simulink model "TailSitter_waypoints_continuous"  (R2018b)
settings: Solver=VariableStepAuto  StartTime=0.0  StopTime=400  RelTol=1e-3
values from neighbouring files (symbols this model uses):
  p =     [ds.mat]    (also in vxs.mat)
undefined symbols (not defined in the file or in its folder): quatnormalize
libraries: aerolibutil x18, simulink x6, sharedutil x3, vrlib x2, simulink_extras x2, sharedtransform x1
(part 1 of 4)
settings Model: Creator=Robert  LastModifiedBy=Robert

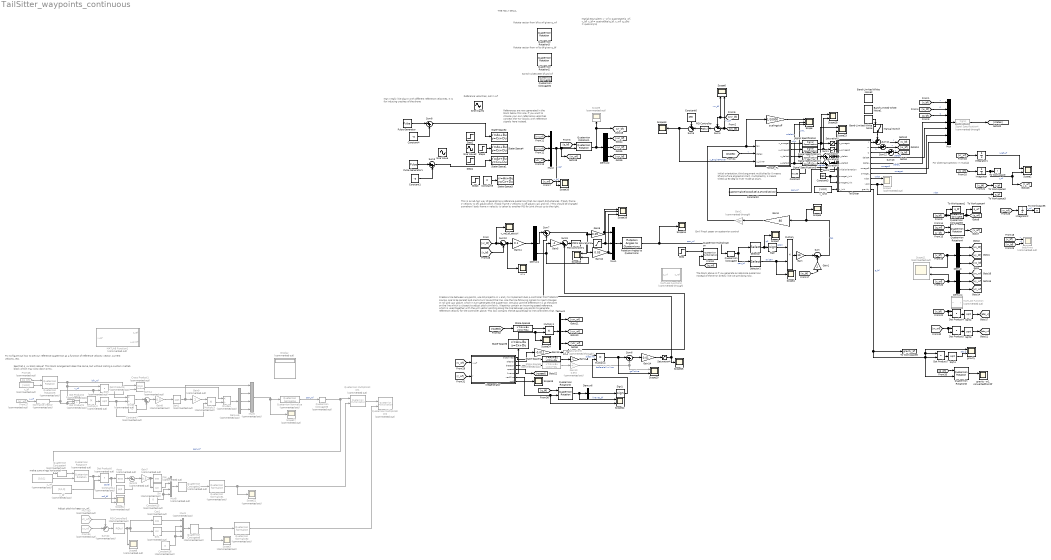
== system TailSitter_waypoints_continuous ==
  note: The block above is if you generate an absolute
      | quaternion instead of the error directy like we are doing now.
  note: References are now generated in the
      |  block below this one. If you want to
      | choose your own referrence velocities
      | connect the "to" blocks with reference
      | signals here instead.
  note: Create a line between waypoints, use 2d projectio in x and y to implement dual p-controller from robotics course, one to be paralell and one to turn toward the line.
      | Use the line following signals to inject changes in roll and yaw above, which in turn generates the quaternion.
      | We also use the difference in z at the point on the line which is closest to adjust pitch similairly.
      | Wapoints contain an incoming speed reference, which is used together with the unit vector pointing along the line between waypoints to generate reference velocity for the
      | controller above. This box contains the be parallell/go to line controllers that modify
      | the above generated signals.
      | I use low pass filters on the line vector and speed to avoid sharp jumps
      | when switching waypoints.
  note: Initial orientation; third argument multiplied
      | by 0 means bf and wf are aligned at start,
      | multiplied by 1 means tilted up 90 deg to
      | hiver mode at start,
  note: Man I really like playin with different reference
      | velocities, it is fun inducing crashes of the drone
  note: This is an ad-hoc way of generating a reference quaternion that can reject disturbances.
      | If body frame z-velocity is off, adjust pitch. If body frame y-velocity is off adjust yaw and roll. (This should be changed somehow)
      | body frame x-velocity is taken by another PID for joint thrust up to the right.
  note: THE HOLY GRAIL
  note: Reference velocities, set in wf
  note: For plotting trajectory in matlab
  note: Emil Fresk paper on quaternion control
  note: Rotate vector from bf to wf given q_wf
  note: Switch q between bf and wf
  note: Rotate vector from wf to bf given q_bf
  note: Matlab equivalent:
      |
      | v_wf = quatrotate(q_wf, v_bf)
      |
      |
      |
      |
      | v_bf = quatrotate(q_bf, v_wf)
      |
      |
      |
      |
      |
      |
      |
      | q_conj = quatconj(q)
  note: Adjust pitch to keep vzr_wf
  note: make sure wings horisontal
  note: See that q_uv block above? This block arangement does the same, but without calling a custom matlab block which may slow down sims.
  note: Try to figure out how to set our reference quaternion as a function of reference velocity vector, current velocity, etc.
  Acos : Trigonometry  Commented=on  Operator=acos
  Band-Limited White Noise : simulink/Sources/Band-Limited White Noise  Cov=[0.01]  Ts=0.2  seed=[23343]
  Band-Limited White Noise1 : simulink/Sources/Band-Limited White Noise  Cov=[0.01]  Ts=0.1  seed=[23342]
  Band-Limited White Noise2 : simulink/Sources/Band-Limited White Noise  Cov=[0.01]  Ts=0.1  seed=[23341]
  Constant : Constant  Value=-0.195
  Constant1 : Constant  Value=-5
  Constant14 : Constant  Commented=on  Value=pi/2
  Constant15 : Constant  Commented=on  Value=0
  Constant16 : Constant  Commented=on  Value=0
  Constant2 : Constant  Value=quatnormalize([cosd(45),0,1*sind(45),0])  VectorParams1D=off
  Constant3 : Constant  Value=290
  Constant4 : Constant  Value=-6
  Constant6 : Constant  Value=290
  Constant7 : Constant  Commented=on
  Constant9 : Constant  Value=0
  Cos : Trigonometry  Commented=on  Operator=cos
  Cos1 : Trigonometry  Commented=on  Operator=cos
  Cross Product1 : vrlib/Utilities/Cross Product  Commented=on
      settings: SourceProductBaseCode=VR
  Demux{,1..4,6} (6 alike) : Demux  Outputs=3
  Demux5 : Demux  Commented=on  Outputs=3
  Display : Display  Commented=on
  Divide : Product  Commented=on  Inputs=*/
  Divide1 : Product  Commented=on  Inputs=*/
  Dot Product{1..3,6} (4 alike) : DotProduct  Commented=on  InputSameDT=on  OutDataTypeStr=Inherit: Inherit via internal rule
  Dot Product4 : DotProduct  InputSameDT=on  OutDataTypeStr=Inherit: Inherit via internal rule
  Dot Product5 : DotProduct  InputSameDT=on  OutDataTypeStr=Inherit: Inherit via internal rule
  Dot Product7 : DotProduct  InputSameDT=on  OutDataTypeStr=Inherit: Inherit via internal rule
  From26 : From  Commented=on  GotoTag=q_wf
  From27 : From  Commented=on  GotoTag=vr_wf
  From33 : From  Commented=on  GotoTag=vz_wf
  From34 : From  Commented=on  GotoTag=vzr_wf
  Gain : Gain  Gain=16
  Gain1 : Gain  Gain=2
  Gain10 : Gain  Commented=on  Gain=0.5*0
  Gain11 : Gain  Gain=0.1
  Gain12 : Gain  Gain=0.03
  Gain13 : Gain  Gain=-0.012
  Gain14 : Gain  Gain=0.01
  Gain2 : Gain  Commented=through  Gain=100
  Gain3 : Gain  Gain=80
  Gain4 : Gain  Gain=-1
  Gain5 : Gain  Gain=-1
  Gain6 : Gain  Gain=0.05
  Gain7 : Gain  Commented=on  Gain=0.5
  Gain8 : Gain  Commented=on  Gain=0.5
  Gain9 : Gain  Commented=on  Gain=2
  Integrator : Integrator
  Integrator1 : Integrator
  Integrator2 : Integrator
  MATLAB Function : MATLAB Function  Commented=on  TreatAsAtomicUnit=on
  MATLAB Function1 : MATLAB Function  Commented=on  TreatAsAtomicUnit=on
  MATLAB Function2 : MATLAB Function  Commented=through  TreatAsAtomicUnit=on
  Manual Switch : ManualSwitch  CurrentSetting=0
  Multiply : Product
  Multiply1 : Product
  Multiply2 : Product  Commented=on
  Multiply3 : Product  Commented=on
  Multiply4 : Product
  Mux : Mux  Inputs=7
  Mux1 : Mux  Inputs=3
  Mux2 : Mux  Inputs=3
  Mux5 : Mux  Commented=on
  Mux8 : Mux  Commented=on
  Mux9 : Mux  Commented=on
  Normalize Vector : vrlib/Utilities/Normalize Vector  Commented=on  maxzero=0
      settings: SourceProductName=Simulink 3D Animation  SourceProductBaseCode=VR
  PID Controller : simulink/Continuous/PID Controller  Controller=PID  Form=Parallel  TimeDomain=Continuous-time  SampleTime=-1  IntegratorMethod=Forward Euler  FilterMethod=Forward Euler  ControllerParametersSource=internal  P=50*3  I=25*2  D=0  UseFilter=on  N=100  TunerSelectOption=Transfer Function Based (PID Tuner App)  InitialConditionSource=internal  InitialConditionForIntegrator=0  InitialConditionForFilter=0  DifferentiatorICPrevScaledInput=0  ExternalReset=none  TrackingMode=off  Kt=1  LimitOutput=on  UpperSaturationLimit=2000-290  LowerSaturationLimit=-290  LinearizeAsGain=on  AntiWindupMode=clamping  Kb=1  POutMin=[]  POutMax=[]  IOutMin=[]  IOutMax=[]  DOutMin=[]  DOutMax=[]  NOutMin=[]  NOutMax=[]  SumOutMin=[]  SumOutMax=[]  SaturationOutMin=[]  SaturationOutMax=[]  PParamMin=[]  PParamMax=[]  IParamMin=[]  IParamMax=[]  DParamMin=[]  DParamMax=[]  NParamMin=[]  NParamMax=[]  KbParamMin=[]  KbParamMax=[]  KtParamMin=[]  KtParamMax=[]  KbOutMin=[]  KbOutMax=[]  KtOutMin=[]  KtOutMax=[]  IntegratorOutMin=[]  IntegratorOutMax=[]  FilterOutMin=[]  FilterOutMax=[]  SumI1OutMin=[]  SumI1OutMax=[]  SumI2OutMin=[]  SumI2OutMax=[]  SumI3OutMin=[]  SumI3OutMax=[]  SumI4OutMin=[]  SumI4OutMax=[]  SumDOutMin=[]  SumDOutMax=[]  DifferentiatorOutMin=[]  DifferentiatorOutMax=[]  FilterDiffOutCoefMin=[]  FilterDiffOutCoefMax=[]  ReciprocalOutMin=[]  ReciprocalOutMax=[]  SumDenOutMin=[]  SumDenOutMax=[]  SumNumOutMin=[]  SumNumOutMax=[]  DivideOutMin=[]  DivideOutMax=[]  IntegratorContinuousStateAttributes=''  IntegratorStateMustResolveToSignalObject=off  IntegratorRTWStateStorageClass=Auto  FilterContinuousStateAttributes=''  FilterStateMustResolveToSignalObject=off  FilterRTWStateStorageClass=Auto  ParallelPVariant=InternalParameters  IdealPVariant=Disabled  IVariant=InternalParameters  DVariant=InternalParameters  IntegratorVariant=Continuous  SatVariant=Enabled  AWVariant=ContClampingParallel  PCopyVariant=Disabled  TRVariant=Disabled  FdbkBlocksVariant=Forward  IdealPFdbkVariant=Disabled  SatFdbkVariant=Disabled  DerivativeFilterVariant=ContFilter  NVariant=InternalParameters  NCopyVariant=Disabled  FilterICVariant=InternalICsFilter  IntegratorICVariant=InternalICs  ExternalResetVariant=Disabled  TRSumVariant=Passthrough  SumFdbkVariant=Disabled  SumVariant=Sum_PID
  PID Controller1 : simulink/Continuous/PID Controller  Controller=PID  Form=Parallel  TimeDomain=Continuous-time  SampleTime=-1  IntegratorMethod=Forward Euler  FilterMethod=Forward Euler  ControllerParametersSource=internal  P=0.08  I=0.005  D=0.04  UseFilter=on  N=100  TunerSelectOption=Transfer Function Based (PID Tuner App)  InitialConditionSource=internal  InitialConditionForIntegrator=0  InitialConditionForFilter=0  DifferentiatorICPrevScaledInput=0  ExternalReset=none  TrackingMode=off  Kt=1  LimitOutput=off  UpperSaturationLimit=inf  LowerSaturationLimit=-inf  LinearizeAsGain=on  AntiWindupMode=none  Kb=1  POutMin=[]  POutMax=[]  IOutMin=[]  IOutMax=[]  DOutMin=[]  DOutMax=[]  NOutMin=[]  NOutMax=[]  SumOutMin=[]  SumOutMax=[]  SaturationOutMin=[]  SaturationOutMax=[]  PParamMin=[]  PParamMax=[]  IParamMin=[]  IParamMax=[]  DParamMin=[]  DParamMax=[]  NParamMin=[]  NParamMax=[]  KbParamMin=[]  KbParamMax=[]  KtParamMin=[]  KtParamMax=[]  KbOutMin=[]  KbOutMax=[]  KtOutMin=[]  KtOutMax=[]  IntegratorOutMin=[]  IntegratorOutMax=[]  FilterOutMin=[]  FilterOutMax=[]  SumI1OutMin=[]  SumI1OutMax=[]  SumI2OutMin=[]  SumI2OutMax=[]  SumI3OutMin=[]  SumI3OutMax=[]  SumI4OutMin=[]  SumI4OutMax=[]  SumDOutMin=[]  SumDOutMax=[]  DifferentiatorOutMin=[]  DifferentiatorOutMax=[]  FilterDiffOutCoefMin=[]  FilterDiffOutCoefMax=[]  ReciprocalOutMin=[]  ReciprocalOutMax=[]  SumDenOutMin=[]  SumDenOutMax=[]  SumNumOutMin=[]  SumNumOutMax=[]  DivideOutMin=[]  DivideOutMax=[]  IntegratorContinuousStateAttributes=''  IntegratorStateMustResolveToSignalObject=off  IntegratorRTWStateStorageClass=Auto  FilterContinuousStateAttributes=''  FilterStateMustResolveToSignalObject=off  FilterRTWStateStorageClass=Auto  ParallelPVariant=InternalParameters  IdealPVariant=Disabled  IVariant=InternalParameters  DVariant=InternalParameters  IntegratorVariant=Continuous  SatVariant=Disabled  AWVariant=Passthrough  PCopyVariant=Disabled  TRVariant=Disabled  FdbkBlocksVariant=Forward  IdealPFdbkVariant=Disabled  SatFdbkVariant=Disabled  DerivativeFilterVariant=ContFilter  NVariant=InternalParameters  NCopyVariant=Disabled  FilterICVariant=InternalICsFilter  IntegratorICVariant=InternalICs  ExternalResetVariant=Disabled  TRSumVariant=Passthrough  SumFdbkVariant=Disabled  SumVariant=Sum_PID
  PID Controller5 : simulink/Continuous/PID Controller  Commented=on  Controller=PID  Form=Parallel  TimeDomain=Continuous-time  SampleTime=-1  IntegratorMethod=Forward Euler  FilterMethod=Forward Euler  ControllerParametersSource=internal  P=0.04*2  I=0  D=0  UseFilter=on  N=100  TunerSelectOption=Transfer Function Based (PID Tuner App)  InitialConditionSource=internal  InitialConditionForIntegrator=0  InitialConditionForFilter=0  DifferentiatorICPrevScaledInput=0  ExternalReset=none  TrackingMode=off  Kt=1  LimitOutput=off  UpperSaturationLimit=inf  LowerSaturationLimit=-inf  LinearizeAsGain=on  AntiWindupMode=none  Kb=1  POutMin=[]  POutMax=[]  IOutMin=[]  IOutMax=[]  DOutMin=[]  DOutMax=[]  NOutMin=[]  NOutMax=[]  SumOutMin=[]  SumOutMax=[]  SaturationOutMin=[]  SaturationOutMax=[]  PParamMin=[]  PParamMax=[]  IParamMin=[]  IParamMax=[]  DParamMin=[]  DParamMax=[]  NParamMin=[]  NParamMax=[]  KbParamMin=[]  KbParamMax=[]  KtParamMin=[]  KtParamMax=[]  KbOutMin=[]  KbOutMax=[]  KtOutMin=[]  KtOutMax=[]  IntegratorOutMin=[]  IntegratorOutMax=[]  FilterOutMin=[]  FilterOutMax=[]  SumI1OutMin=[]  SumI1OutMax=[]  SumI2OutMin=[]  SumI2OutMax=[]  SumI3OutMin=[]  SumI3OutMax=[]  SumI4OutMin=[]  SumI4OutMax=[]  SumDOutMin=[]  SumDOutMax=[]  DifferentiatorOutMin=[]  DifferentiatorOutMax=[]  FilterDiffOutCoefMin=[]  FilterDiffOutCoefMax=[]  ReciprocalOutMin=[]  ReciprocalOutMax=[]  SumDenOutMin=[]  SumDenOutMax=[]  SumNumOutMin=[]  SumNumOutMax=[]  DivideOutMin=[]  DivideOutMax=[]  IntegratorContinuousStateAttributes=''  IntegratorStateMustResolveToSignalObject=off  IntegratorRTWStateStorageClass=Auto  FilterContinuousStateAttributes=''  FilterStateMustResolveToSignalObject=off  FilterRTWStateStorageClass=Auto  ParallelPVariant=InternalParameters  IdealPVariant=Disabled  IVariant=InternalParameters  DVariant=InternalParameters  IntegratorVariant=Continuous  SatVariant=Disabled  AWVariant=Passthrough  PCopyVariant=Disabled  TRVariant=Disabled  FdbkBlocksVariant=Forward  IdealPFdbkVariant=Disabled  SatFdbkVariant=Disabled  DerivativeFilterVariant=ContFilter  NVariant=InternalParameters  NCopyVariant=Disabled  FilterICVariant=InternalICsFilter  IntegratorICVariant=InternalICs  ExternalResetVariant=Disabled  TRSumVariant=Passthrough  SumFdbkVariant=Disabled  SumVariant=Sum_PID
  Pulse Generator : DiscretePulseGenerator  PulseType=Time based  Amplitude=12  Period=50  PulseWidth=50
  Pulse Generator1 : DiscretePulseGenerator  PulseType=Time based  Amplitude=8  Period=60  PulseWidth=50  PhaseDelay=30
  Quaternion Conjugate : aerolibutil/Quaternion Conjugate
      settings: SourceProductName=Aerospace Blockset  SourceProductBaseCode=AE
  Quaternion Conjugate{1,4..6} (4 alike) : aerolibutil/Quaternion Conjugate  Commented=on
      settings: SourceProductName=Aerospace Blockset  SourceProductBaseCode=AE
  Quaternion Conjugate2 : aerolibutil/Quaternion Conjugate
      settings: SourceProductName=Aerospace Blockset  SourceProductBaseCode=AE
  Quaternion Conjugate3 : aerolibutil/Quaternion Conjugate
      settings: SourceProductName=Aerospace Blockset  SourceProductBaseCode=AE
  Quaternion Multiplication : aerolibutil/Quaternion Multiplication
  Quaternion Multiplication1 : aerolibutil/Quaternion Multiplication  Commented=on
  Quaternion Multiplication2 : aerolibutil/Quaternion Multiplication  Commented=on
  Quaternion Normalize : sharedutil/Quaternion Normalize  Commented=on  aMode=aMode
      settings: SourceProductName=Aerospace Blockset  SourceProductBaseCode=AE
  Quaternion Normalize1 : sharedutil/Quaternion Normalize  Commented=on  aMode=aMode
      settings: SourceProductName=Aerospace Blockset  SourceProductBaseCode=AE
  Quaternion Normalize2 : sharedutil/Quaternion Normalize  Commented=on  aMode=aMode
      settings: SourceProductName=Aerospace Blockset  SourceProductBaseCode=AE
  Quaternion Rotation{1..4,6,8} (6 alike) : aerolibutil/Quaternion Rotation
  Quaternion Rotation5 : aerolibutil/Quaternion Rotation  Commented=on
  Quaternion Rotation7 : aerolibutil/Quaternion Rotation  Commented=on
  Rotation Angles to Quaternions : sharedtransform/Rotation Angles to Quaternions  rotationOrder=ZYX  aMode=aMode
      settings: SourceProductName=Aerospace Blockset  SourceProductBaseCode=AE
  Saturation : Saturate  UpperLimit=1000  LowerLimit=0
  Saturation1 : Saturate  UpperLimit=1000  LowerLimit=0
  Saturation2 : Saturate  UpperLimit=1  LowerLimit=-1
  Saturation3 : Saturate  UpperLimit=1  LowerLimit=-1
  Saturation4 : Saturate
  Saturation5 : Saturate  Commented=through  UpperLimit=1  LowerLimit=-1
  Saturation6 : Saturate
  Scope : Scope  NumInputPorts=3
  Scope1 : Scope  Commented=on  NumInputPorts=2
  Scope{2,6,10,15,18,20,22..23} (8 alike) : Scope  NumInputPorts=2
  Scope11 : Scope  Commented=on  NumInputPorts=2
  Scope12 : Scope  Commented=on  NumInputPorts=2
  Scope{4..5,7,13..14,19,24..25} (8 alike) : Scope
  Scope16 : Scope  NumInputPorts=3
  Scope{3,8..9,17,21} (5 alike) : Scope  Commented=on
  Selector : Selector  IndexMode=Zero-based  InputPortWidth=4  IndexOptions=Index vector (dialog)  Indices=[0 ]  OutputSizes=1
  Selector1 : Selector  IndexMode=Zero-based  InputPortWidth=4  IndexOptions=Index vector (dialog)  Indices=[1:3]  OutputSizes=1
  Sign : Signum
  Sign1 : Signum
  Signal Specification{,1..3} (4 alike) : SignalSpecification  Dimensions=1
  Signal Specification4 : SignalSpecification  Commented=through  Dimensions=14
  Sin : Trigonometry  Commented=on
  Sin1 : Trigonometry  Commented=on
  Sine Wave : Sin  Amplitude=-2  Frequency=1/15  Phase=pi/2  SampleTime=0
  Sine Wave1 : Sin  Amplitude=-8  Frequency=1/20  SampleTime=0
  Sine Wave2 : Sin  Amplitude=10  Frequency=1/45  SampleTime=0
  Sqrt : Sqrt  Commented=on  SaturateOnIntegerOverflow=on
  Sqrt1 : Sqrt  Commented=on  SaturateOnIntegerOverflow=on
  Sqrt2 : Sqrt  SaturateOnIntegerOverflow=on
  Sqrt3 : Sqrt  SaturateOnIntegerOverflow=on
  Sqrt4 : Sqrt  SaturateOnIntegerOverflow=on
  State-Space1 : StateSpace  A=-1/5  B=1/5  D=0  InitialCondition=0
  State-Space2 : StateSpace  A=-1/15  B=1/15  D=0  InitialCondition=0
  State-Space3 : StateSpace  A=-1/15  B=1/15  D=0  InitialCondition=0
  State-Space4 : StateSpace  A=-1/15  B=1/15  D=0  InitialCondition=0
  State-Space5 : StateSpace  A=-1/5  B=1/5  D=0  InitialCondition=0
  State-Space6 : StateSpace  A=-1/2*eye(3)  B=1/2*eye(3)  C=eye(3)  D=0*eye(3)  InitialCondition=0
  State-Space7 : StateSpace  A=-1/4  B=1/4  D=0  InitialCondition=0
  State-Space8 : StateSpace  Commented=on  A=-1/15  B=1/15  D=0  InitialCondition=0
  Step : Step  Time=15  Before=quatnormalize([cosd(45),0,1*sind(45),0])  After=quatnormalize([cosd(30),0,1*sind(30),0])  SampleTime=0
  Step1 : Step  Time=20  After=-10  SampleTime=0
  Step2 : Step  Time=100  After=5  SampleTime=0
  Step3 : Step  Time=30  Before=-1  After=0  SampleTime=0
  Step4 : Step  Time=60  After=18  SampleTime=0
  Sum : Sum  Inputs=|--
  Sum{1..3,7..9} (6 alike) : Sum  Inputs=|++
  Sum10 : Sum  Inputs=|+-
  Sum{5,11..13} (4 alike) : Sum  Inputs=++|
  Sum14 : Sum  Commented=on  Inputs=|++
  Sum21 : Sum  Commented=on  Inputs=|+-
  Sum22 : Sum  Commented=on  Inputs=-+|
  Sum4 : Sum  Inputs=+-|
  Sum6 : Sum  Inputs=|-+
  TailSitter : Subsystem
  To Workspace : ToWorkspace  VariableName=r  SaveFormat=Timeseries  SampleTime=p.Ts
  To Workspace1 : ToWorkspace  VariableName=q_bf  SaveFormat=Timeseries  SampleTime=0.5
  To Workspace2 : ToWorkspace  VariableName=v_bf  SaveFormat=Timeseries  SampleTime=p.Ts
  To Workspace3 : ToWorkspace  VariableName=a_bf  SaveFormat=Timeseries  SampleTime=p.Ts
  To Workspace4 : ToWorkspace  VariableName=q_wf  SaveFormat=Timeseries  SampleTime=p.Ts
  To Workspace5 : ToWorkspace  VariableName=rr  SaveFormat=Timeseries  SampleTime=p.Ts
  To Workspace6 : ToWorkspace  VariableName=gravity_bf  SaveFormat=Timeseries  SampleTime=p.Ts
  Torque_FL : MATLAB Function  TreatAsAtomicUnit=on
  bodyfrme : Scope  Commented=on  NumInputPorts=2
  gravity : Scope  NumInputPorts=2
  gravity_wf_convertedfrombf : Scope  NumInputPorts=2
  linegenerator : MATLAB Function  TreatAsAtomicUnit=on
  scalingstuff : Gain  Gain=1/10000
  v_isnit : Constant  Value=[1,0,0]
  "v_ref_bf_attctrl " : Scope
  vr-v : Scope
  x_bf : Constant  Commented=on  Value=[1,0,0]
  y_bf : Constant  Commented=on  Value=[0,1,0]
  z_wf : Constant  Commented=on  Value=[0,0,1]
  wires:
  [q_wf] -> Quaternion Multiplication/2
  Quaternion Conjugate/1 -> Selector/1, Selector1/1  "qerr_bf"
  Selector1/1 -> Scope4/1, Multiply/2  "axiserr"
  Selector/1 -> Scope7/1, Sign/1  "q0"
  Sign/1 -> Multiply/1  "rotdir"
  Gain1/1 -> Sum/2
  Sum5/1 -> Torque_FL/3(u_jointT), Scope13/1  "u_EnginePower"
  Constant3/1 -> TailSitter/7(omegaR_init), TailSitter/6(omegaL_init)
  Sum11/1 -> [v_bf]  "v"
  TailSitter/8(wdot) -> Scope1/1  "wdot"
  TailSitter/9(vdot) -> To Workspace3/1, Scope1/2  "vdot"
  Integrator/1 -> [r_wf], Scope2/2, To Workspace/1  "r_wf"
  [v_wf] -> Integrator/1
  v_isnit/1 -> TailSitter/8(v_init)
  Sum4/1 -> PID Controller/1
  Sum/1 -> Scope5/1, Gain3/1  "tao"
  PID Controller/1 -> Sum5/2
  Constant6/1 -> Sum5/1
  Multiply/1 -> Gain/1
  [vxr_bf] -> Sum4/1, Scope6/1  "vxr_bf"
  Saturation/1 -> TailSitter/2(u_omegaR)
  Saturation1/1 -> TailSitter/1(u_omegaL)
  TailSitter/3(q) -> Sum13/2
  Mux2/1 -> Scope10/2, [vr_wf], Quaternion Rotation1/2  "vref"
  Quaternion Rotation1/1 -> Demux2/1, [vr_bf], Scope9/1
  Demux2/3 -> [vzr_bf]
  Demux2/2 -> [vyr_bf]
  Demux2/1 -> [vxr_bf]
  [vx_bf] -> Scope6/2, Sum4/2  "vx_bf"
  [v_wf] -> Scope10/1  "v_wf"
  [q_bf] -> Quaternion Rotation1/1
  [q_bf] -> To Workspace1/1, Quaternion Conjugate3/1
  Quaternion Conjugate3/1 -> To Workspace4/1, [q_wf]
  [vxr_wf] -> Mux2/1
  [vyr_wf] -> Mux2/2
  [vzr_wf] -> Mux2/3
  [q_wf] -> Quaternion Rotation4/1
  Quaternion Rotation4/1 -> [v_wf]
  [v_bf] -> Quaternion Rotation4/2
  TailSitter/2(w) -> Sum12/2  "w"
  Demux/1 -> [vx_bf]
  Demux/3 -> [vz_bf]
  Demux/2 -> [vy_bf]
  [v_bf] -> Scope11/1, Demux/1
  Demux4/2 -> [vy_wf]
  Demux4/3 -> [vz_wf]
  Demux4/1 -> [vx_wf]
  [v_wf] -> Scope11/2, Demux4/1
  [v_bf] -> To Workspace2/1
  [v_bf] -> Dot Product4/2, Dot Product4/1
  Sqrt2/1 -> [abs_v]
  [vr_wf] -> Integrator1/1
  Integrator1/1 -> Scope2/1  "r_ref_wf"
  [w_bf] -> Gain1/1
  [v_bf] -> bodyfrme/1  "v"
  [vr_bf] -> bodyfrme/2  "vr"
  [vr_wf] -> Integrator2/1
  Integrator2/1 -> To Workspace5/1  "r_wf"
  Dot Product4/1 -> Sqrt2/1
  Gain/1 -> Sum/1
  Constant2/1 -> TailSitter/5(initialOrientation)  "qerr_wf"
  [v_bf] -> Mux/1  "v"
  [w_bf] -> Mux/2  "w"
  [q_bf] -> Mux/3  "q"
  TailSitter/5(deltaL) -> Mux/4  "deltaL"
  TailSitter/4(deltaR) -> Mux/5  "deltaR"
  TailSitter/7(omegaL) -> Mux/6  "omegaL"
  TailSitter/6(omegaR) -> Mux/7  "omegaR"
  Torque_FL/1(u_omegaL) -> Signal Specification/1  "uWL"
  Torque_FL/2(u_omegaR) -> Signal Specification1/1
  Torque_FL/3(u_deltaL) -> Scope/2, Signal Specification2/1  "uWL"
  Torque_FL/4(u_deltaR) -> Signal Specification3/1, Scope/3  "udeltaL"
  Signal Specification/1 -> Scope18/1, Saturation1/1
  Signal Specification1/1 -> Scope18/2, Saturation/1
  Signal Specification2/1 -> Sum1/1
  Signal Specification3/1 -> Sum2/1
  Mux/1 -> Signal Specification4/1
  Sum1/1 -> Saturation2/1
  [states] -> Torque_FL/2(states)  "v"
  Signal Specification4/1 -> [states]
  Gain3/1 -> Gain2/1
  scalingstuff/1 -> Scope/1
  Acos/1 -> Sum21/1
  y_bf/1 -> Dot Product6/2
  Multiply3/1 -> Divide1/2
  Sum22/1 -> PID Controller5/1
  Dot Product3/1 -> Divide/1
  Demux5/2 -> Mux5/3
  Quaternion Conjugate6/1 -> Scope3/1, Quaternion Normalize2/1
  Mux5/1 -> Scope17/1, Quaternion Normalize/1
  From33/1 -> Sum22/1
  Constant15/1 -> Mux8/3, Mux8/4
  Mux8/1 -> Quaternion Conjugate1/1
  Demux5/1 -> Mux5/2
  PID Controller5/1 -> Scope8/1, Cos1/1, Sin1/1
  From27/1 -> Normalize Vector/1  "v_wf"
  Cos1/1 -> Mux9/1
  Quaternion Rotation7/1 -> Scope12/1, Dot Product6/1  "zwf_bf"
  Constant16/1 -> Mux9/2, Mux9/4
  Quaternion Normalize1/1 -> Scope21/1, Quaternion Multiplication1/2
  Gain7/1 -> Sin/1, Cos/1
  Sum21/1 -> Gain7/1
  From34/1 -> Sum22/2
  Mux9/1 -> Quaternion Conjugate6/1
  Cos/1 -> Mux8/1
  Constant14/1 -> Sum21/2
  Sin/1 -> Mux8/2
  Quaternion Normalize2/1 -> Quaternion Multiplication2/2
  Multiply2/1 -> Sqrt/1
  Divide/1 -> Sum14/1
  Quaternion Conjugate1/1 -> Quaternion Normalize1/1
  Sin1/1 -> Mux9/3
  Sqrt1/1 -> Mux5/1, Gain9/1
  Quaternion Conjugate4/1 -> Quaternion Rotation7/1
  Normalize Vector/1 -> Cross Product1/2, Dot Product3/2, Dot Product2/1, Dot Product2/2  "v_wf"
  Quaternion Normalize/1 -> Quaternion Conjugate5/1  "qerr_wf"
  Gain8/1 -> Sqrt1/1
  Cross Product1/1 -> Divide1/1
  Divide1/1 -> Demux5/1
  From26/1 -> Quaternion Rotation5/1
  Sum14/1 -> Gain8/1
  z_wf/1 -> Quaternion Rotation7/2
  Dot Product6/1 -> Scope12/2, Acos/1  "cos(a)"
  Gain9/1 -> Multiply3/1
  Dot Product1/1 -> Multiply2/1
  Constant7/1 -> Sum14/2
  Dot Product2/1 -> Multiply2/2
  Sqrt/1 -> Multiply3/2, Divide/2
  Quaternion Rotation5/1 -> Dot Product3/1, Dot Product1/2, Dot Product1/1, Cross Product1/1  "bfx_wf"
  Demux5/3 -> Mux5/4
  x_bf/1 -> Quaternion Rotation5/2
  Quaternion Multiplication1/1 -> Quaternion Multiplication2/1
  Quaternion Conjugate5/1 -> Quaternion Conjugate4/1, Quaternion Multiplication1/1  "qerr_wf"
  Mux1/1 -> Rotation Angles to Quaternions/1
  [v_bf] -> Sum10/2
  Sum10/1 -> vr-v/1, Gain11/1
  Demux1/3 -> Gain5/1, Scope15/2
  Gain5/1 -> Sum9/1
  Sum7/1 -> Gain12/1, Gain6/1
  Gain6/1 -> Scope16/1, Mux1/1
  PID Controller1/1 -> Saturation6/1, Scope15/1
  Gain11/1 -> Demux1/1
  Saturation2/1 -> Scope23/1, TailSitter/3(u_deltaL)
  Sum2/1 -> Saturation3/1
  Saturation3/1 -> Scope23/2, TailSitter/4(u_deltaR)
  Constant/1 -> Sum2/2, Sum1/2  "udeltaL"
  Sum3/1 -> State-Space1/1
  Gain12/1 -> Mux1/3, Scope16/3
  Dot Product5/1 -> Sqrt3/1
  Sqrt3/1 -> [abs_vr]
  [vr_wf] -> Dot Product5/2, Dot Product5/1
  [vr_bf] -> "v_ref_bf_attctrl "/1, Sum10/1
  Sum8/1 -> State-Space2/1
  Step4/1 -> State-Space4/1
  TailSitter/10(gravity) -> To Workspace6/1, gravity/1, Dot Product7/1, Quaternion Rotation8/2, Dot Product7/2  "g_bf"
  Dot Product7/1 -> Sqrt4/1
  [q_wf] -> Quaternion Rotation8/1
  Quaternion Rotation8/1 -> gravity_wf_convertedfrombf/1
  Pulse Generator1/1 -> Sum3/1
  Constant1/1 -> Sum3/2
  Pulse Generator/1 -> Sum8/1
  Constant4/1 -> Sum8/2
  Sqrt4/1 -> gravity/2  "abs g"
  Gain2/1 -> scalingstuff/1, Torque_FL/1(tao)
  Step/1 -> Quaternion Multiplication/1
  [v_wf] -> linegenerator/1(v_wf)
  linegenerator/1(dist2line2d) -> State-Space7/1
  linegenerator/3(thetaerr) -> State-Space8/1
  Gain4/1 -> Multiply4/1  "dist2line"
  Gain10/1 -> Scope20/1, Sum6/2  "beParalell w line"
  [r_wf] -> linegenerator/2(r)
  linegenerator/4(rspeed) -> [rspeed]
  [rspeed] -> State-Space5/1
  linegenerator/5(linevec) -> State-Space6/1
  Demux3/1 -> [vxr_wf]
  Multiply1/1 -> Demux3/1
  Demux1/2 -> Sum7/1
  Sum6/1 -> Gain14/1
  linegenerator/2(altError) -> Gain13/1
  Gain13/1 -> Saturation5/1
  linegenerator/7(wpN) -> Scope19/1
  Demux3/2 -> [vyr_wf]
  Demux3/3 -> [vzr_wf]
  Gain14/1 -> Saturation4/1
  [q_bf] -> Quaternion Rotation6/1
  Quaternion Rotation6/1 -> Scope22/1, Demux6/1  "linevec_bf"
  Sign1/1 -> Multiply4/2
  Multiply4/1 -> Scope20/2, Sum6/1  "goToLine"
  Sum9/1 -> PID Controller1/1
  linegenerator/6(vec2line) -> Scope22/2, Quaternion Rotation6/2
  Demux6/2 -> Sign1/1
  Saturation4/1 -> Scope25/1, Sum7/2
  Saturation5/1 -> Sum9/2
  State-Space6/1 -> Scope24/1, Multiply1/2
  State-Space5/1 -> Multiply1/1
  State-Space7/1 -> Gain4/1
  State-Space8/1 -> Gain10/1
  Saturation6/1 -> Scope16/2, Mux1/2
  Constant9/1 -> State-Space3/1
  TailSitter/1(v) -> Sum11/2  "v"
  Sum12/1 -> [w_bf]  "v"
  Sum13/1 -> [q_bf]  "v"
  Band-Limited White Noise/1 -> Manual Switch/1
  Manual Switch/1 -> Sum11/1
  Rotation Angles to Quaternions/1 -> Scope14/1, Quaternion Conjugate/1  "qerr_wf"

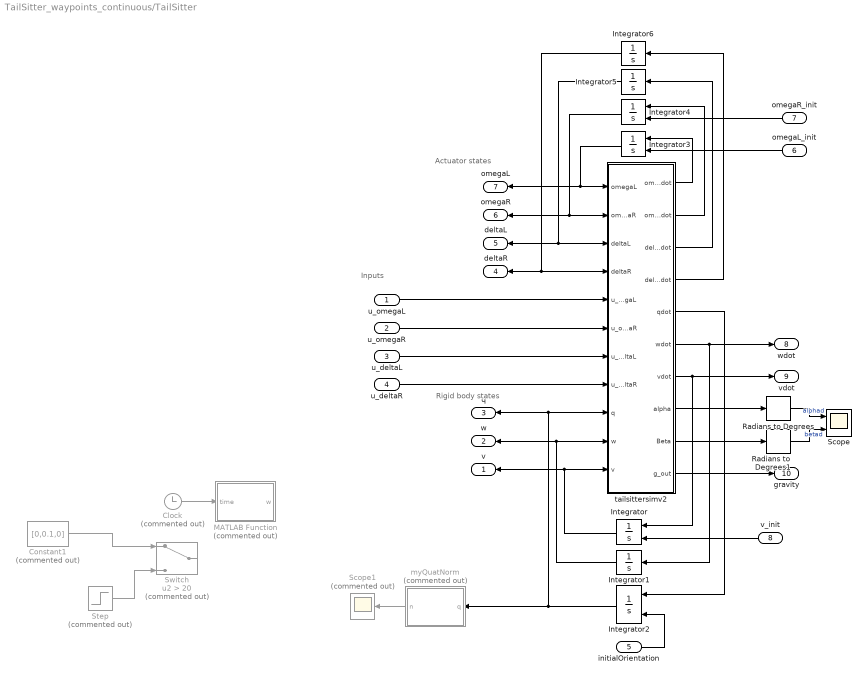
== system TailSitter_waypoints_continuous/TailSitter ==
  note: Actuator
      | states
  note: Rigid
      | body
      | states
  note: Inputs
  u_omegaL : Inport
  u_omegaR : Inport  Port=2
  u_deltaL : Inport  Port=3
  u_deltaR : Inport  Port=4
  initialOrientation : Inport  Port=5
  omegaL_init : Inport  Port=6
  omegaR_init : Inport  Port=7
  v_init : Inport  Port=8
  Clock : Clock  Commented=on
  Constant1 : Constant  Commented=on  Value=[0,0.1,0]
  Integrator : Integrator  InitialConditionSource=external  InitialCondition=[0,0,0]
  Integrator1 : Integrator  InitialCondition=[0,0,0]
  Integrator2 : Integrator  InitialConditionSource=external
  Integrator3 : Integrator  InitialConditionSource=external
  Integrator4 : Integrator  InitialConditionSource=external
  Integrator5 : Integrator
  Integrator6 : Integrator
  MATLAB Function : MATLAB Function  Commented=on  TreatAsAtomicUnit=on
  Radians to Degrees : simulink_extras/Transformations/Radians to Degrees
  Radians to Degrees1 : simulink_extras/Transformations/Radians to Degrees
  Scope : Scope  NumInputPorts=2
  Scope1 : Scope  Commented=on
  Step : Step  Commented=on  Time=10  Before=[0.1,0,0]  After=[0,0,0.1]  SampleTime=0
  Switch : Switch  Commented=on  Criteria=u2 > Threshold  Threshold=20
  myQuatNorm : MATLAB Function  Commented=on  TreatAsAtomicUnit=on
  tailsittersimv2 : MATLAB Function  TreatAsAtomicUnit=on
  v : Outport
  w : Outport  Port=2
  q : Outport  Port=3
  deltaR : Outport  Port=4
  deltaL : Outport  Port=5
  omegaR : Outport  Port=6
  omegaL : Outport  Port=7
  wdot : Outport  Port=8  PortDimensions=3
  vdot : Outport  Port=9  PortDimensions=3
  gravity : Outport  Port=10  PortDimensions=3
  wires:
  tailsittersimv2/7(vdot) -> Integrator/1, vdot/1
  tailsittersimv2/6(wdot) -> Integrator1/1, wdot/1
  tailsittersimv2/5(qdot) -> Integrator2/1
  Integrator2/1 -> tailsittersimv2/9(q), q/1, myQuatNorm/1(q)
  initialOrientation/1 -> Integrator2/2
  tailsittersimv2/1(omegaLdot) -> Integrator3/1
  Integrator3/1 -> tailsittersimv2/1(omegaL), omegaL/1
  tailsittersimv2/2(omegaRdot) -> Integrator4/1
  tailsittersimv2/3(deltaLdot) -> Integrator5/1
  tailsittersimv2/4(deltaRdot) -> Integrator6/1
  Integrator5/1 -> tailsittersimv2/3(deltaL), deltaL/1
  Integrator6/1 -> tailsittersimv2/4(deltaR), deltaR/1
  Integrator4/1 -> tailsittersimv2/2(omegaR), omegaR/1
  omegaL_init/1 -> Integrator3/2
  omegaR_init/1 -> Integrator4/2
  u_omegaL/1 -> tailsittersimv2/5(u_omegaL)
  u_omegaR/1 -> tailsittersimv2/6(u_omegaR)
  u_deltaL/1 -> tailsittersimv2/7(u_deltaL)
  u_deltaR/1 -> tailsittersimv2/8(u_deltaR)
  tailsittersimv2/8(alpha) -> Radians to Degrees/1
  Radians to Degrees/1 -> Scope/1  "alphad"
  myQuatNorm/1(n) -> Scope1/1
  Integrator/1 -> tailsittersimv2/11(v), v/1
  Clock/1 -> MATLAB Function/1(time)
  Constant1/1 -> Switch/1
  Step/1 -> Switch/3
  Integrator1/1 -> tailsittersimv2/10(w), w/1
  v_init/1 -> Integrator/2
  tailsittersimv2/9(Beta) -> Radians to Degrees1/1
  Radians to Degrees1/1 -> Scope/2  "betad"
  tailsittersimv2/10(g_out) -> gravity/1
